simulink model "c_pend"  (Simulink 6.3)
settings: Solver=ode23tb  StartTime=0.0  StopTime=20.0  RelTol=1e-3
values from neighbouring files (symbols this model uses):
  Cp = [ alf1    0   0 ... (first row only)    [init_c_pend.m]    (also in init_d_pend.m; mod_pend.m)
  gd1 = 1.080    (= 1.08)    [act_pend.m]    (also in init_c_pend.m; init_d_pend.m)
  gd2 = 0.335    [act_pend.m]    (also in init_c_pend.m; init_d_pend.m)
  kf = 0.00002    (= 2e-05)    [init_c_pend.m]    (also in init_d_pend.m)
  Td1 = 0.005    [act_pend.m]    (also in init_c_pend.m; init_d_pend.m)
  Td2 = 0.002    [act_pend.m]    (also in init_c_pend.m; init_d_pend.m)
  Tf1 = 10    [init_c_pend.m]    (also in init_d_pend.m)
  Tf2 = 0.1    [init_c_pend.m]    (also in init_d_pend.m)
undefined symbols (not defined in the file or in its folder): Ak, Bk, Ck, Dk
libraries: simulink x3
settings Model: LastModifiedBy=Petko Petkov  StrictBusMsg=None
settings DataIOCC: SignalLoggingName=sigsOut
settings OptimizationCC: BooleanDataType=off  InlineInvariantSignals=on
settings DebuggingCC: SolverPrmCheckMsg=none
settings HardwareCC: TargetUnknown=on
settings GRTTargetCC: ModelReferenceCompliant=off  MatFileLogging=off

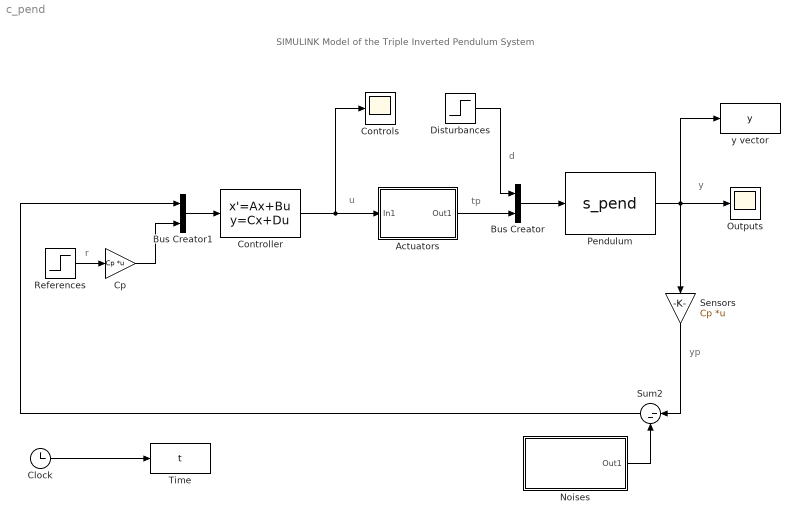
== system c_pend ==
  note: SIMULINK Model of the Triple Inverted Pendulum System
  note: r
  note: yp
  note: u
  note: d
  note: tp
  note: y
  Actuators : Subsystem
  Bus Creator : BusCreator  Inputs=2
  Bus Creator1 : BusCreator  Inputs=2
  Clock : Clock
  Controller : StateSpace  A=Ak  B=Bk  C=Ck  D=Dk
  Controls : Scope
      settings: YMin=-0.225  YMax=0.15  MaxDataPoints=10000
  Cp : Gain  Gain=Cp  Multiplication=Matrix(K*u)  SaturateOnIntegerOverflow=on
  Disturbances : Step  Time=0  Before="[0  0  0]"  After="[0  0  0]"  SampleTime=0
  Noises : Subsystem
  Outputs : Scope
      settings: YMin=-0.1  YMax=0.75  MaxDataPoints=10000
  Pendulum : S-Function  FunctionName=s_pend
  References : Step  Time=0  Before="[0  0  0]"  After="[0  -0.1  0.2]"  SampleTime=0
  Sensors : Gain  Orientation=down  Gain=Cp  Multiplication=Matrix(K*u)  SaturateOnIntegerOverflow=on
  Sum2 : Sum  Orientation=left  Inputs=|--  SaturateOnIntegerOverflow=on  InputSameDT=on
  Time : ToWorkspace  VariableName=t  SampleTime=-1  SaveFormat=Array
  y vector : ToWorkspace  VariableName=y  SampleTime=-1  SaveFormat=Array
  wires:
  References/1 -> Cp/1
  Bus Creator/1 -> Pendulum/1
  Controller/1 -> Controls/1, Actuators/1(In1)
  Disturbances/1 -> Bus Creator/1
  Sum2/1 -> Bus Creator1/1
  Noises/1(Out1) -> Sum2/2
  Actuators/1(Out1) -> Bus Creator/2
  Pendulum/1 -> Outputs/1, Sensors/1, y vector/1
  Sensors/1 -> Sum2/1
  Cp/1 -> Bus Creator1/2
  Bus Creator1/1 -> Controller/1
  Clock/1 -> Time/1

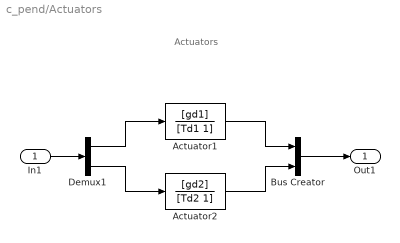
== system c_pend/Actuators ==
  note: Actuators
  In1 : Inport
  Actuator1 : TransferFcn  Numerator=[gd1]  Denominator=[Td1 1]
  Actuator2 : TransferFcn  Numerator=[gd2]  Denominator=[Td2 1]
  Bus Creator : BusCreator  Inputs=2
  Demux1 : Demux  Outputs=[1, 1]
  Out1 : Outport
  wires:
  In1/1 -> Demux1/1
  Demux1/1 -> Actuator1/1
  Demux1/2 -> Actuator2/1
  Actuator1/1 -> Bus Creator/1
  Actuator2/1 -> Bus Creator/2
  Bus Creator/1 -> Out1/1

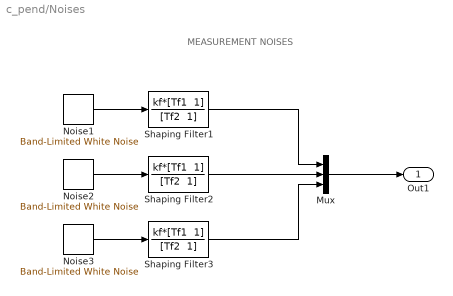
== system c_pend/Noises ==
  note: MEASUREMENT NOISES
  Mux : Mux  Inputs=3
  Noise1 : simulink/Sources/Band-Limited White Noise  Cov=10^(-4)  Ts=0.1  seed=[23341]
  Noise2 : simulink/Sources/Band-Limited White Noise  Cov=10^(-4)  Ts=0.1  seed=[57456]
  Noise3 : simulink/Sources/Band-Limited White Noise  Cov=10^(-4)  Ts=0.1  seed=[79865]
  Shaping Filter1 : TransferFcn  Numerator="kf*[Tf1  1]"  Denominator="[Tf2  1]"
  Shaping Filter2 : TransferFcn  Numerator="kf*[Tf1  1]"  Denominator="[Tf2  1]"
  Shaping Filter3 : TransferFcn  Numerator="kf*[Tf1  1]"  Denominator="[Tf2  1]"
  Out1 : Outport
  wires:
  Mux/1 -> Out1/1
  Noise1/1 -> Shaping Filter1/1
  Noise2/1 -> Shaping Filter2/1
  Noise3/1 -> Shaping Filter3/1
  Shaping Filter1/1 -> Mux/1
  Shaping Filter2/1 -> Mux/2
  Shaping Filter3/1 -> Mux/3
